simulink model "ADAS_Main"  (R2026a)
settings: Solver=FixedStepDiscrete  StopTime=5
InitFcn:
  | createLidarActorProfiles;
model workspace (MAT data in the model file):
  firstWarning = 1
  originalScenarioChecksum = '71EAF3DF157DF5A35F75811B676F8B0F'
undefined symbols (not defined in the file): driving, matlabshared
libraries: drivingscenarioandsensors x3, lidarlib x1
(part 5 of 6)

== matlab function ADAS_Main/Behavior_Planning/Plan_Feasibility ==
  data: CandV input; CandFeasStatus output; CandCurv input; CandValid input; CandFeasible output; CandViolFlags output; CandPeakAy output; CandKappa output; CandPeakDemand output; CandExceedsEmergency output; CandPeakLatJerk output; CandExceedsLateralJerk output; HardValid output; NormalValid output; ConfigFault output
function [CandFeasStatus, CandFeasible, CandViolFlags, CandPeakAy, CandKappa, ...
          CandPeakDemand, CandExceedsEmergency, CandPeakLatJerk, ...
          CandExceedsLateralJerk, HardValid, NormalValid, ConfigFault] = ...
    Plan_Feasibility(CandV, CandCurv, CandValid) %#codegen
%PLAN_FEASIBILITY  Planning Stage 2 - DYNAMIC FEASIBILITY ONLY.
%
%   Determines whether each of the 35 Stage-1 candidates is dynamically
%   feasible. It performs NO collision checking, NO risk evaluation, NO
%   manoeuvre selection and NO planning decision.
%
%   It reads ONLY the candidate trajectory and configured vehicle/ODD
%   parameters. No TrackState, TrackID, TrackCov, TrackAttributes, Verdict3,
%   RiskValid, M_adm or Bind is available to it - that independence is
%   structural, not conventional, because no such input is wired.
%
%   NOTE ON HORIZONS: every equation below is evaluated per SAMPLE and none
%   requires a time value, so Stage 2 introduces NO horizon grid of its own.
%   It consumes the existing Stage-1 35 x 11 sample structure unchanged.
%
% HARD constraints - these and only these reject a candidate
%   H2   |kappa| <= KAPPA_MAX                      once per candidate
%   H3a  ax      <= A_ACC_MAX                      once per candidate
%   H4'  sqrt(ax^2 + ay^2) <= MU_LO*G              ALL 11 samples
%        with ay = v^2 * kappa      (no division by v anywhere)
%
% NORMAL constraints - DIAGNOSTIC ONLY, never reject
%   N1   |ay| <= A_Y_NORMAL
%   N2   |ax| <= A_BRK_NORMAL       not evaluated while A_BRK_NORMAL is unset
%
% DIAGNOSTIC ONLY - never reject, never alter CandFeasStatus
%   lateral jerk  j_y = 2*v*ax*kappa      (trajectory diagnostic; NO claim of
%                 regulatory equivalence to a half-second moving average)
%   emergency     |ax| >= EmergencyBoundary
%
% H2 and H3a are evaluated once per candidate because kappa and ax are constant
% by construction in Stage 1 (measured: max |kappa(n+1)-kappa(n)| = 0.000e+00).
% The test suite asserts per-sample evaluation is bit-identical, so the
% assumption is monitored rather than trusted.

%% ---- constants, copied VERBATIM from plan_par.m ------------------------
MAXC = 35;
NH   = 11;
G    = 9.80665;
ACC_TABLE = [-8.0 -5.0 -1.0 0.0 2.0];

% Vehicle geometry (B) and the declared turning assumption (E). KAPPA_MAX is
% DERIVED here with the identical expression used in plan_par.m rather than
% written as a decimal literal: a 15-digit literal does not round-trip and
% would differ from plan_par.m by 1 ulp, breaking the single-source discipline.
% Deriving it makes the two bit-identical by construction.
L_WB   = 2.80;                   % B  wheelbase [m]
W_VEH  = 1.80;                   % B  overall body width [m]
FO_VEH = 0.90;                   % B  front overhang [m]
R_WALL_DECLARED = 6.0;           % E  DECLARED RESEARCH-MODEL ASSUMPTION [m]
R_r       = sqrt(R_WALL_DECLARED^2 - (L_WB + FO_VEH)^2) - W_VEH/2;   % F
KAPPA_MAX = 1/R_r;                                                    % F
A_ACC_MAX = 2.0;                 % E  DECLARED RESEARCH-MODEL ASSUMPTION
MU_LO     = 0.50;                % E  DECLARED RESEARCH-MODEL ASSUMPTION

A_Y_NORMAL        = 3.0;         % C  provisional, UN R79 - diagnostic only
A_BRK_NORMAL      = NaN;         %    UNRESOLVED / non-blocking
LateralJerkNormal = 5.0;         % C  provisional, UN R79 - diagnostic only
EmergencyBoundary = 6.0;         % C  UN R13-H - diagnostic only

%% ---- parameter validity: gate on the FLAG, never on the value ----------
% The only permitted read of a parameter that may be unset is the finiteness
% and positivity test that establishes its invalidity. No NaN ever reaches a
% constraint comparison, because every comparison is guarded by its flag.
MU_VALID           = isfinite(MU_LO)             && (MU_LO > 0);
KAPPA_VALID        = isfinite(KAPPA_MAX)         && (KAPPA_MAX > 0);
AACC_VALID         = isfinite(A_ACC_MAX)         && (A_ACC_MAX > 0);
AY_NORMAL_VALID    = isfinite(A_Y_NORMAL)        && (A_Y_NORMAL > 0);
ABRK_NORMAL_VALID  = isfinite(A_BRK_NORMAL)      && (A_BRK_NORMAL > 0);
JERK_NORMAL_VALID  = isfinite(LateralJerkNormal) && (LateralJerkNormal > 0);

HardValid   = MU_VALID && KAPPA_VALID && AACC_VALID;
NormalValid = AY_NORMAL_VALID && ABRK_NORMAL_VALID;
ConfigFault = ~HardValid;        % NORMAL validity never contributes

MU_LIMIT = 0;
if MU_VALID
    MU_LIMIT = MU_LO*G;
end

%% ---- outputs preallocated ---------------------------------------------
CandFeasStatus         = zeros(MAXC,1,'int8');
CandFeasible           = false(MAXC,1);
CandViolFlags          = zeros(MAXC,1,'uint8');
CandPeakAy             = zeros(MAXC,1);
CandKappa              = zeros(MAXC,1);
CandPeakDemand         = zeros(MAXC,1);
CandExceedsEmergency   = false(MAXC,1);
CandPeakLatJerk        = zeros(MAXC,1);
CandExceedsLateralJerk = false(MAXC,1);

for c = 1:MAXC
    if ~CandValid(c)
        % not generated: definitively not executable; all diagnostics zero
        CandFeasStatus(c) = int8(2);
        CandViolFlags(c)  = uint8(1);
        if ~HardValid
            CandViolFlags(c) = bitor(CandViolFlags(c), uint8(64));
        end
        continue
    end

    ia = floor((c-1)/7) + 1;
    ax = ACC_TABLE(ia);
    k  = CandCurv(c,1);
    CandKappa(c) = k;

    peakAy = 0; peakDem = 0; peakJerk = 0;
    h4ok = true; n1ok = true;
    for n = 1:NH
        v  = CandV(c,n);
        kk = CandCurv(c,n);
        ay = v*v*kk;
        if abs(ay) > peakAy, peakAy = abs(ay); end
        dem = sqrt(ax*ax + ay*ay);
        if dem > peakDem, peakDem = dem; end
        jy = 2*v*ax*kk;
        if abs(jy) > peakJerk, peakJerk = abs(jy); end
        if MU_VALID && dem > MU_LIMIT,        h4ok = false; end
        if AY_NORMAL_VALID && abs(ay) > A_Y_NORMAL, n1ok = false; end
    end
    CandPeakAy(c)      = peakAy;
    CandPeakDemand(c)  = peakDem;
    CandPeakLatJerk(c) = peakJerk;

    h2ok = true;
    if KAPPA_VALID && abs(k) > KAPPA_MAX, h2ok = false; end
    h3ok = true;
    if AACC_VALID && ax > A_ACC_MAX, h3ok = false; end
    n2ok = true;
    if ABRK_NORMAL_VALID && abs(ax) > A_BRK_NORMAL, n2ok = false; end

    f = uint8(0);
    if KAPPA_VALID && ~h2ok, f = bitor(f,uint8(2));  end
    if AACC_VALID  && ~h3ok, f = bitor(f,uint8(4));  end
    if MU_VALID    && ~h4ok, f = bitor(f,uint8(8));  end
    if AY_NORMAL_VALID   && ~n1ok, f = bitor(f,uint8(16)); end
    if ABRK_NORMAL_VALID && ~n2ok, f = bitor(f,uint8(32)); end
    if ~HardValid,                 f = bitor(f,uint8(64)); end
    CandViolFlags(c) = f;

    % NORMAL bits 16/32 and the diagnostics below appear NOWHERE in evalFail.
    evalFail = (KAPPA_VALID && ~h2ok) || (AACC_VALID && ~h3ok) || (MU_VALID && ~h4ok);
    if evalFail
        CandFeasStatus(c) = int8(2);
    elseif HardValid
        CandFeasStatus(c) = int8(1);
    else
        CandFeasStatus(c) = int8(0);
    end

    if JERK_NORMAL_VALID && peakJerk > LateralJerkNormal
        CandExceedsLateralJerk(c) = true;
    end
    if abs(ax) >= EmergencyBoundary
        CandExceedsEmergency(c) = true;
    end
end

CandFeasible = (CandFeasStatus == int8(1));
end

== matlab function ADAS_Main/Behavior_Planning/Plan_Envelopes ==
  data: CandX input; CandSpatialStatus output; CandY input; CandCurv input; CandFeasStatus input; TrackState input; TrackAttributes input; TrackStatus input; TrackID input; CandMinSeparation output; CandFirstConflictH output; CandConflictCount output; CandConflictIDs output; CandSpatialFlags output; NumSpatialFeasible output
function [CandSpatialStatus, CandMinSeparation, CandFirstConflictH, ...
          CandConflictCount, CandConflictIDs, CandSpatialFlags, ...
          NumSpatialFeasible] = Plan_Envelopes( ...
          CandX, CandY, CandCurv, CandFeasStatus, ...
          TrackState, TrackAttributes, TrackStatus, TrackID) %#codegen
%PLAN_ENVELOPES  Planning Stage 3 - SPATIAL / ENVELOPE FEASIBILITY ONLY.
%
%   Answers: does each Stage-2 FEASIBLE candidate stay spatially clear of the
%   predicted tracked environment over the approved horizons?
%
%   It is NOT risk scoring, NOT manoeuvre selection, NOT behaviour or intention
%   inference, NOT TTC, and NOT a second fusion stage. It produces per-candidate
%   spatial evidence; Risk and Stage 4 consume it. TrackCov is deliberately NOT
%   an input - uncertainty stays in the Risk Engine.
%
%   STATELESS. No Unit Delay, no Memory, no persistent. Every cycle evaluates
%   all current candidates against the current environment.
%
% PREDICTION (approved): Prediction_Horizons propagates the mean with a constant
%   velocity model, so the predicted mean is exactly p + v*h. Verified against
%   the logged trkPred over 51 frames x 7 horizons at max difference 0.000e+00.
%   TrackPredictions is therefore NOT exposed from Tracking and no new Planning
%   input is required. The test suite asserts this identity permanently.
%
% LIMITATION, recorded deliberately: Stage 3 is SAMPLED spatial feasibility at
%   7 horizons, NOT a continuous collision guarantee. Between consecutive
%   samples 0.5 s elapses, during which a 15 m/s closing speed covers 7.5 m.
%   Swept-volume checking is not implemented. This is not minimised.

%% ---- constants, copied VERBATIM from plan_par.m ------------------------
MAXC = 35; MAXT = 512; MAXREJ = 32; NHS = 7;
HS   = [0.5 1.0 1.5 2.0 3.0 4.0 5.0];
HIDX = [2 3 4 5 7 9 11];

EGO_BOX_XMIN = -1.00; EGO_BOX_XMAX = 3.70;
EGO_BOX_YMIN = -0.90; EGO_BOX_YMAX = 0.90;
PLANNING_EGO_COLLISION_MARGIN = 0.0;
OBJECT_ORIENTATION_SPEED_THRESHOLD = 1.0;
SEP_NOOBJ = 1000.0;

% ego collision box, expressed about the rear-axle reference point
EGO_CX = 0.5*(EGO_BOX_XMIN + EGO_BOX_XMAX);                            % 1.35
EGO_HX = 0.5*(EGO_BOX_XMAX - EGO_BOX_XMIN) + PLANNING_EGO_COLLISION_MARGIN;
EGO_HY = 0.5*(EGO_BOX_YMAX - EGO_BOX_YMIN) + PLANNING_EGO_COLLISION_MARGIN;

%% ---- outputs preallocated ---------------------------------------------
CandSpatialStatus  = zeros(MAXC,1,'int8');
CandMinSeparation  = SEP_NOOBJ*ones(MAXC,NHS);
CandFirstConflictH = zeros(MAXC,1,'uint8');
CandConflictCount  = zeros(MAXC,1,'uint16');
CandConflictIDs    = zeros(MAXC,MAXREJ,'uint32');
CandSpatialFlags   = zeros(MAXC,1,'uint8');
NumSpatialFeasible = uint16(0);

seen = false(MAXT,1);

for c = 1:MAXC
    % Stage-2 rejection is ABSORBING: a candidate the vehicle cannot execute
    % can never become feasible through good clearance.
    if CandFeasStatus(c) ~= int8(1)
        CandSpatialStatus(c) = int8(2);
        CandSpatialFlags(c)  = uint8(1);
        continue
    end

    for t = 1:MAXT, seen(t) = false; end
    nConf = uint16(0); overflow = false;
    anyOverlap = false; anyUnknown = false;
    firstH = uint8(0);
    fUnusable = false; fDims = false; fCoast = false;

    for hi = 1:NHS
        n = HIDX(hi);
        h = HS(hi);
        kap = CandCurv(c,n);
        cx  = CandX(c,n);
        cy  = CandY(c,n);
        % ego heading on the constant-curvature arc: kap*x = sin(psi),
        % 1 - kap*y = cos(psi). Exact, and atan2(0,1) = 0 when kap = 0.
        psi = atan2(kap*cx, 1 - kap*cy);
        cp  = cos(psi); sp = sin(psi);
        eEx = cp; eEy = sp;                 % ego longitudinal axis
        fEx = -sp; fEy = cp;                % ego lateral axis
        ecx = cx + EGO_CX*cp;               % ego box centre
        ecy = cy + EGO_CX*sp;

        minsep = SEP_NOOBJ;
        for t = 1:MAXT
            if TrackStatus(t) == 0
                continue                     % FREE slot: not an object
            end
            if TrackAttributes(t,1) ~= 1
                anyUnknown = true; fUnusable = true; continue
            end
            Lo = TrackAttributes(t,2);
            Wo = TrackAttributes(t,3);
            if ~isfinite(Lo) || ~isfinite(Wo) || Lo <= 0 || Wo <= 0
                anyUnknown = true; fDims = true; continue
            end
            px = TrackState(t,1); py = TrackState(t,2);
            vx = TrackState(t,3); vy = TrackState(t,4);
            if ~isfinite(px) || ~isfinite(py) || ~isfinite(vx) || ~isfinite(vy)
                anyUnknown = true; continue
            end
            ocx = px + vx*h;                 % approved prediction: p + v*h
            ocy = py + vy*h;
            if ~isfinite(ocx) || ~isfinite(ocy)
                anyUnknown = true; continue
            end
            if TrackStatus(t) == 3
                fCoast = true;
            end

            sv = sqrt(vx*vx + vy*vy);
            if sv > OBJECT_ORIENTATION_SPEED_THRESHOLD
                oEx = vx/sv; oEy = vy/sv;    % oriented along velocity
            else
                oEx = 1.0;  oEy = 0.0;       % axis-aligned fallback
            end
            oFx = -oEy; oFy = oEx;
            ohx = 0.5*Lo; ohy = 0.5*Wo;

            dx = ocx - ecx; dy = ocy - ecy;

            % separating-axis test over the 4 box axes
            sep = -realmax;
            for ax = 1:4
                if ax == 1
                    axx = eEx; axy = eEy;
                elseif ax == 2
                    axx = fEx; axy = fEy;
                elseif ax == 3
                    axx = oEx; axy = oEy;
                else
                    axx = oFx; axy = oFy;
                end
                rE = abs(EGO_HX*(axx*eEx + axy*eEy)) + abs(EGO_HY*(axx*fEx + axy*fEy));
                rO = abs(ohx *(axx*oEx + axy*oEy)) + abs(ohy *(axx*oFx + axy*oFy));
                d  = abs(dx*axx + dy*axy);
                g  = d - (rE + rO);
                if g > sep, sep = g; end
            end

            if sep < minsep, minsep = sep; end

            if sep <= 0
                anyOverlap = true;
                if firstH == uint8(0), firstH = uint8(hi); end
                if ~seen(t)
                    seen(t) = true;
                    nConf = nConf + uint16(1);
                    if nConf <= uint16(MAXREJ)
                        CandConflictIDs(c,double(nConf)) = TrackID(t);
                    else
                        overflow = true;
                    end
                end
            end
        end
        CandMinSeparation(c,hi) = minsep;
    end

    CandConflictCount(c)  = nConf;           % ALL conflicts, never truncated
    CandFirstConflictH(c) = firstH;

    f = uint8(0);
    if anyOverlap, f = bitor(f,uint8(2));  end
    if fUnusable,  f = bitor(f,uint8(4));  end
    if fDims,      f = bitor(f,uint8(8));  end
    if fCoast,     f = bitor(f,uint8(16)); end
    if overflow,   f = bitor(f,uint8(32)); end
    CandSpatialFlags(c) = f;

    % A definite overlap is certifiable even when unknowns are present, so
    % INFEASIBLE takes precedence over UNKNOWN. Uncertainty is never converted
    % into safety: an unusable track leaves the candidate UNKNOWN, not FEASIBLE.
    if anyOverlap
        CandSpatialStatus(c) = int8(2);
    elseif anyUnknown
        CandSpatialStatus(c) = int8(0);
    else
        CandSpatialStatus(c) = int8(1);
        NumSpatialFeasible = NumSpatialFeasible + uint16(1);
    end
end
end

== matlab function ADAS_Main/Behavior_Planning/Plan_Evaluate ==
  data: CandY input; CandAdmissible output; CandV input; CandFeasStatus input; CandSpatialStatus input; CandMinSeparation input; EgoKinematics input; CandWorstClearance output; CandLateralOffset output; CandSpeedDelta output; CandRejectReason output
function [CandAdmissible, CandWorstClearance, CandLateralOffset, ...
          CandSpeedDelta, CandRejectReason] = Plan_Evaluate( ...
          CandY, CandV, CandFeasStatus, CandSpatialStatus, ...
          CandMinSeparation, EgoKinematics) %#codegen
%PLAN_EVALUATE  Planning Stage 4a - per-candidate comparative metrics.
%
%   Computes the quantities the lexicographic selector needs. It performs NO
%   selection, NO ranking, NO risk evaluation, NO TTC, NO intention inference
%   and NO behaviour classification.
%
%   STATELESS. No Unit Delay, no Memory, no persistent.
%
%   HARD GATE, and the only one:
%       admissible(c) = (CandFeasStatus(c) == 1) AND (CandSpatialStatus(c) == 1)
%   A candidate must pass BOTH Stage 2 and Stage 3 to be selectable. Note that
%   NumFeasible (Stage-2 count) is NOT the number of selectable candidates.
%
%   ICE and Risk are deliberately absent from this block. They are indexed by
%   sector x horizon, not by candidate, and are never reinterpreted as
%   candidate scores.

MAXC = 35; NHS = 7;

CandAdmissible     = false(MAXC,1);
CandWorstClearance = zeros(MAXC,1);
CandLateralOffset  = zeros(MAXC,1);
CandSpeedDelta     = zeros(MAXC,1);
CandRejectReason   = zeros(MAXC,1,'uint8');

v0 = EgoKinematics(1);
if ~isfinite(v0), v0 = 0; end
if v0 < 0, v0 = 0; end

for c = 1:MAXC
    % terminal-sample metrics are defined for every candidate, admissible or not
    CandLateralOffset(c) = CandY(c,11);
    CandSpeedDelta(c)    = abs(CandV(c,11) - v0);

    wc = CandMinSeparation(c,1);
    for h = 2:NHS
        if CandMinSeparation(c,h) < wc, wc = CandMinSeparation(c,h); end
    end
    CandWorstClearance(c) = wc;

    adm = (CandFeasStatus(c) == int8(1)) && (CandSpatialStatus(c) == int8(1));
    CandAdmissible(c) = adm;

    % rejection reason, retained for ALL 35 candidates and never truncated.
    % 'not selected' (8) is applied later by Plan_Select; here an admissible
    % candidate carries 0 until selection resolves it.
    if CandFeasStatus(c) ~= int8(1)
        CandRejectReason(c) = uint8(1);          % Stage-2 rejection
    elseif CandSpatialStatus(c) == int8(2)
        CandRejectReason(c) = uint8(2);          % Stage-3 overlap
    elseif CandSpatialStatus(c) == int8(0)
        CandRejectReason(c) = uint8(4);          % Stage-3 unknown
    else
        CandRejectReason(c) = uint8(0);
    end
end
end

== matlab function ADAS_Main/Behavior_Planning/Plan_Select ==
  data: CandAdmissible input; TrajX output; CandWorstClearance input; CandLateralOffset input; CandSpeedDelta input; CandRejectReason input; CandX input; CandY input; CandV input; CandCurv input; CandFeasStatus input; CandSpatialStatus input; TrackStatus input; ConfigFault input; RiskValid input; TrajY output; TrajV output; TrajCurv output; TrajValid output; ManoeuvreLabel output; FallbackActive output; NumFeasible output; NumClear output; NumTracksEvaluated output; RejectIDs output; PlanStale output; NoFeasibleReason output; RejectOverflow output; SelectedCandidate output; CandRejectReasonOut output
function [TrajX, TrajY, TrajV, TrajCurv, TrajValid, ManoeuvreLabel, ...
          FallbackActive, NumFeasible, NumClear, NumTracksEvaluated, ...
          RejectIDs, PlanStale, NoFeasibleReason, RejectOverflow, ...
          SelectedCandidate, CandRejectReasonOut] = Plan_Select( ...
          CandAdmissible, CandWorstClearance, CandLateralOffset, ...
          CandSpeedDelta, CandRejectReason, ...
          CandX, CandY, CandV, CandCurv, ...
          CandFeasStatus, CandSpatialStatus, TrackStatus, ...
          ConfigFault, RiskValid) %#codegen
%PLAN_SELECT  Planning Stage 4b - lexicographic selection and public outputs.
%
%   STATELESS. No Unit Delay, no Memory, no persistent, no previous-selection
%   state. Every cycle selects from the CURRENT admissible set only, so an
%   ongoing manoeuvre has no privileged status: if the candidate selected last
%   cycle is no longer admissible it simply is not in the set. There is no
%   overtaking mode, no abort mode, no "obstacle handled" state, and no
%   primary-object priority.
%
% HARD GATE - the only selection path
%   admissible(c) = (CandFeasStatus(c)==1) AND (CandSpatialStatus(c)==1)
%   INVARIANT: TrajValid == true  =>  both hold for the selected candidate.
%
% LEXICOGRAPHIC ORDER with tolerance bands (no weighted sum, no score)
%   KEY 1  CandWorstClearance  larger preferred   band BAND_CLEAR = 0.05 m
%   KEY 2  |CandLateralOffset| smaller preferred  band BAND_LAT   = 0.50 m
%   KEY 3  CandSpeedDelta      smaller preferred  band BAND_SPD   = 2.50 m/s
%   TIE    lowest candidate index
%   CandProgress is NOT a ranking key: forward distance may never buy down
%   clearance.
%
% ZERO-FEASIBLE STATE
%   FallbackActive = true means "Planning has no admissible trajectory and is
%   NOT commanding one". It does NOT mean emergency braking is commanded. No
%   fallback manoeuvre exists in the current candidate library and none is
%   fabricated here.

MAXC = 35; NH = 11; MAXREJ = 32; MAXT = 512;

% tolerance bands, copied VERBATIM from plan_par.m
BAND_CLEAR = 0.05;
BAND_LAT   = 0.50;
BAND_SPD   = 2.50;

TrajX  = zeros(NH,1); TrajY = zeros(NH,1);
TrajV  = zeros(NH,1); TrajCurv = zeros(NH,1);
TrajValid          = false;
ManoeuvreLabel     = uint8(0);
FallbackActive     = false;
NumFeasible        = uint16(0);
NumClear           = uint16(0);
NumTracksEvaluated = uint16(0);
RejectIDs          = zeros(MAXREJ,1,'uint32');
PlanStale          = false;
NoFeasibleReason   = uint8(0);
RejectOverflow     = false;
SelectedCandidate  = uint8(0);
CandRejectReasonOut = CandRejectReason;

%% ---- counts ------------------------------------------------------------
nS2 = uint16(0); nS3 = uint16(0);
for c = 1:MAXC
    if CandFeasStatus(c) == int8(1),    nS2 = nS2 + uint16(1); end
    if CandSpatialStatus(c) == int8(1), nS3 = nS3 + uint16(1); end
end
NumFeasible = nS2;      % Stage-2 count. NOT the number of selectable candidates.
NumClear    = nS3;      % Stage-3 count.
nT = uint16(0);
for t = 1:MAXT
    if TrackStatus(t) ~= 0, nT = nT + uint16(1); end
end
NumTracksEvaluated = nT;

%% ---- PlanStale: input usability only, NOT "nothing is feasible" -------
% AdmVacuous is deliberately excluded: it is an ICE scene state, not a
% statement that a Planning input is unusable.
PlanStale = ConfigFault || ~RiskValid;

%% ---- KEY 1: worst-case clearance, larger preferred ---------------------
nAdm = 0; best1 = 0;
for c = 1:MAXC
    if CandAdmissible(c)
        if nAdm == 0 || CandWorstClearance(c) > best1, best1 = CandWorstClearance(c); end
        nAdm = nAdm + 1;
    end
end

if nAdm == 0
    FallbackActive = true;
    TrajValid      = false;          % never true without an admissible candidate
    ManoeuvreLabel = uint8(0);
    if PlanStale
        NoFeasibleReason = uint8(8);                 % upstream invalid
    elseif nS2 == uint16(0)
        NoFeasibleReason = uint8(1);                 % all rejected at Stage 2
    elseif nS2 == uint16(MAXC)
        NoFeasibleReason = uint8(2);                 % all rejected at Stage 3
    else
        NoFeasibleReason = uint8(4);                 % mixed
    end
else
    keep1 = false(MAXC,1);
    for c = 1:MAXC
        if CandAdmissible(c) && CandWorstClearance(c) >= best1 - BAND_CLEAR
            keep1(c) = true;
        end
    end

    % KEY 2: |lateral offset|, smaller preferred
    best2 = 0; first = true;
    for c = 1:MAXC
        if keep1(c)
            a = abs(CandLateralOffset(c));
            if first || a < best2, best2 = a; first = false; end
        end
    end
    keep2 = false(MAXC,1);
    for c = 1:MAXC
        if keep1(c) && abs(CandLateralOffset(c)) <= best2 + BAND_LAT
            keep2(c) = true;
        end
    end

    % KEY 3: terminal-speed disturbance, smaller preferred
    best3 = 0; first = true;
    for c = 1:MAXC
        if keep2(c)
            if first || CandSpeedDelta(c) < best3, best3 = CandSpeedDelta(c); first = false; end
        end
    end
    keep3 = false(MAXC,1);
    for c = 1:MAXC
        if keep2(c) && CandSpeedDelta(c) <= best3 + BAND_SPD
            keep3(c) = true;
        end
    end

    % TIE: lowest candidate index
    sel = 0;
    for c = 1:MAXC
        if keep3(c), sel = c; break; end
    end

    SelectedCandidate = uint8(sel);
    ManoeuvreLabel    = uint8(sel);          % the candidate index IS the label
    TrajValid         = true;
    FallbackActive    = false;
    for n = 1:NH
        TrajX(n)    = CandX(sel,n);
        TrajY(n)    = CandY(sel,n);
        TrajV(n)    = CandV(sel,n);
        TrajCurv(n) = CandCurv(sel,n);
    end
    CandRejectReasonOut(sel) = uint8(0);
end

%% ---- rejection bookkeeping --------------------------------------------
% every non-selected candidate carries a reason; admissible-but-not-selected
% is reason 8. Nothing is silently discarded.
for c = 1:MAXC
    if uint8(c) ~= SelectedCandidate && CandRejectReasonOut(c) == uint8(0)
        CandRejectReasonOut(c) = uint8(8);
    end
end
nRej = 0;
for c = 1:MAXC
    if CandRejectReasonOut(c) ~= uint8(0)
        nRej = nRej + 1;
        if nRej <= MAXREJ
            RejectIDs(nRej) = uint32(c);     % ascending, deterministic
        else
            RejectOverflow = true;
        end
    end
end
end

== matlab function ADAS_Main/Behavior_Planning/Plan_Continuity ==
  data: CandAdmissible input; TrajX output; CandWorstClearance input; CandX input; CandY input; CandV input; CandCurv input; Challenger input; CandRejectReason input; NumFeasible_in input; NumClear_in input; NumTracksEvaluated_in input; PlanStale_in input; PrevSelected_in input uint8 size=1; SelectionAge_in input uint16 size=1; TrajY output; TrajV output; TrajCurv output; TrajValid output; ManoeuvreLabel output; FallbackActive output; NumFeasible output; NumClear output; NumTracksEvaluated output; RejectIDs output; PlanStale output; PrevSelected_out output; SelectionAge_out output; ContinuityHeld output; SwitchReason output
function [TrajX, TrajY, TrajV, TrajCurv, TrajValid, ManoeuvreLabel, ...
          FallbackActive, NumFeasible, NumClear, NumTracksEvaluated, ...
          RejectIDs, PlanStale, ...
          PrevSelected_out, SelectionAge_out, ContinuityHeld, SwitchReason] = ...
    Plan_Continuity( ...
          CandAdmissible, CandWorstClearance, CandX, CandY, CandV, CandCurv, ...
          Challenger, CandRejectReason, NumFeasible_in, NumClear_in, ...
          NumTracksEvaluated_in, PlanStale_in, PrevSelected_in, SelectionAge_in) %#codegen
%PLAN_CONTINUITY  Planning Stage 5 - temporal continuity / hysteresis.
%
%   Prefers the previously selected candidate while it REMAINS ADMISSIBLE and
%   the current challenger is not materially better. It performs no evaluation,
%   no ranking, no risk assessment and no object reasoning.
%
%   SCENARIO INDEPENDENT BY CONSTRUCTION. Its entire input set is an
%   admissibility mask, one scalar metric per candidate, the challenger index
%   and its own previous index. It cannot see actor IDs, actor counts, object
%   classes, coordinates, road geometry, timing or ego speed, so it cannot
%   contain scenario-specific logic. There is no overtaking mode, no abort
%   mode, no object priority and no "obstacle handled" state.
%
% SAFETY PRIORITY, absolute
%   HARD SAFETY FEASIBILITY  >  TEMPORAL CONTINUITY  >  SOFT PREFERENCE
%   The previous candidate is re-gated against the CURRENT admissibility mask
%   every cycle. Continuity can only ever choose among candidates that are
%   admissible NOW, so it can never make an inadmissible candidate selectable.
%
% NO minimum hold time. NO N-cycle persistence. NO switching penalty or score.
% NO hidden delay. A materially safer challenger replaces the previous
% candidate on the SAME cycle, and an inadmissible previous candidate is
% abandoned on the SAME cycle.

MAXC = 35; NH = 11; MAXREJ = 32;
SWITCH_MARGIN = 0.05;            % copied VERBATIM from plan_par.m

TrajX = zeros(NH,1); TrajY = zeros(NH,1);
TrajV = zeros(NH,1); TrajCurv = zeros(NH,1);
TrajValid          = false;
ManoeuvreLabel     = uint8(0);
FallbackActive     = false;
NumFeasible        = NumFeasible_in;
NumClear           = NumClear_in;
NumTracksEvaluated = NumTracksEvaluated_in;
RejectIDs          = zeros(MAXREJ,1,'uint32');
PlanStale          = PlanStale_in;
ContinuityHeld     = false;
SwitchReason       = uint8(0);
SelectionAge_out   = uint16(0);

%% ---- previous selection, re-gated against the CURRENT mask -------------
prev = PrevSelected_in;
if PlanStale_in
    prev = uint8(0);                 % never rest continuity on unusable input
    SwitchReason = uint8(8);
end
prevOK = false;
if prev ~= uint8(0) && prev <= uint8(MAXC)
    if CandAdmissible(double(prev))
        prevOK = true;               % admissible THIS cycle, not last cycle
    end
end

%% ---- continuity decision -----------------------------------------------
% SWITCH_MARGIN = 0 disables hysteresis entirely, so Stage 5 reproduces
% Stage-4 output bit-identically. The guard is required because Stage 4's
% winner is the LEXICOGRAPHIC winner, which may carry lower clearance than an
% admissible previous candidate; a clearance-only test at margin 0 would still
% retain the previous one and would not reproduce Stage 4.
sel = Challenger;
if (SWITCH_MARGIN > 0) && prevOK
    takeChallenger = false;
    if Challenger ~= uint8(0)
        if CandWorstClearance(double(Challenger)) > ...
           CandWorstClearance(double(prev)) + SWITCH_MARGIN
            takeChallenger = true;   % materially better
        end
    end
    if takeChallenger
        sel = Challenger;
        SwitchReason = uint8(2);
    else
        sel = prev;                  % retained; it passed the gate this cycle
        ContinuityHeld = true;
    end
else
    if SwitchReason == uint8(0)
        if prev == uint8(0)
            SwitchReason = uint8(4); % no previous selection
        elseif ~prevOK
            SwitchReason = uint8(1); % previous no longer admissible
        else
            SwitchReason = uint8(2); % challenger taken (hysteresis disabled)
        end
    end
end

%% ---- emit ---------------------------------------------------------------
rr = CandRejectReason;
if sel ~= uint8(0)
    % defensive: emit ONLY a candidate that passes the current hard gate
    if ~CandAdmissible(double(sel))
        sel = uint8(0);
    end
end

if sel == uint8(0)
    TrajValid        = false;
    FallbackActive   = true;
    ManoeuvreLabel   = uint8(0);
    PrevSelected_out = uint8(0);
    SelectionAge_out = uint16(0);
    for c = 1:MAXC
        if rr(c) == uint8(0), rr(c) = uint8(8); end
    end
else
    TrajValid      = true;
    FallbackActive = false;
    ManoeuvreLabel = sel;
    for n = 1:NH
        TrajX(n)    = CandX(double(sel),n);
        TrajY(n)    = CandY(double(sel),n);
        TrajV(n)    = CandV(double(sel),n);
        TrajCurv(n) = CandCurv(double(sel),n);
    end
    PrevSelected_out = sel;
    if sel == PrevSelected_in && ~PlanStale_in
        SelectionAge_out = SelectionAge_in + uint16(1);
    else
        SelectionAge_out = uint16(1);
    end
    % reject bookkeeping follows the ACTUAL selection, not Stage-4's proposal
    if Challenger ~= uint8(0) && Challenger ~= sel
        rr(double(Challenger)) = uint8(8);
    end
    rr(double(sel)) = uint8(0);
end

nRej = 0;
for c = 1:MAXC
    if rr(c) ~= uint8(0)
        nRej = nRej + 1;
        if nRej <= MAXREJ
            RejectIDs(nRej) = uint32(c);
        end
    end
end
end

== matlab function ADAS_Main/Radar_Perception/Radar_Feature_Extraction/Extract_Radar_Features ==
  data: u input; RadarFeatures output
function RadarFeatures = fcn(u)

N = 50;

RadarFeatures = zeros(N,8);

for i = 1:N
    RadarFeatures(i,1) = double(i <= u.NumDetections);
    RadarFeatures(i,2:7) = double(u.Detections(i).Measurement);
    RadarFeatures(i,8) = double(u.Detections(i).ObjectAttributes.SNR);
end

== matlab function ADAS_Main/Behavior_Controller/Ctrl_Lateral ==
  data: TrajCurv input; SteerCmd output; TrajValid input; EgoKinematics input; CmdValid output; CtrlCurvatureRef output; CtrlState output
function [SteerCmd, CmdValid, CtrlCurvatureRef, CtrlState] = ...
    Ctrl_Lateral(TrajCurv, TrajValid, EgoKinematics) %#codegen
%CTRL_LATERAL  Controller Stage C1 - LATERAL FEEDFORWARD ONLY.
%
%   Converts the curvature of the Planning-selected trajectory into a
%   front-road-wheel-equivalent steering command. It does NOTHING else.
%
% NOT IMPLEMENTED IN C1, BY AUTHORIZATION
%   no longitudinal control, no feedback of any kind (k_y, k_psi, k_v,
%   Stanley, Pure Pursuit, LQR, MPC), no steering-rate limit, no actuator
%   model, no braking or fallback policy, no PlanStale handling, no vehicle
%   dynamics. There is NO state: no persistent, no Unit Delay, no Memory.
%   The block is a pure function of its inputs.
%
% SCENARIO INDEPENDENT BY CONSTRUCTION
%   The entire input set is one curvature array, one boolean, and two ego
%   self-kinematic scalars. The block never receives actor IDs, track IDs,
%   object classes, actor counts, coordinates, road or intersection geometry,
%   lane boundaries or scenario timing, so it cannot contain scenario-specific
%   logic. EgoKinematics is accepted to honour the approved C1 interface and
%   is DELIBERATELY NOT READ - see EGO SPEED below.
%
% EGO SPEED
%   The feedforward law depends on curvature and wheelbase ONLY. Speed does
%   not appear in the kinematic bicycle steering relation. EgoKinematics is
%   therefore left unread, which makes independence from the 15 m/s fixture
%   speed STRUCTURAL rather than a property that has to be tested for.
%
% THE LAW
%   TrajValid == true                        TrajValid == false
%     kappa = TrajCurv(1)                      SteerCmd         = 0
%     d     = atan(L_WB*kappa)                 CmdValid         = false
%     SteerCmd = sat(d, +/-DELTA_MAX)          CtrlCurvatureRef = 0
%     CmdValid = true                          CtrlState        = NO_TRAJECTORY
%     CtrlCurvatureRef = kappa                 (NO trajectory element is read)
%     CtrlState = TRACKING
%
% WHY TrajCurv(1)
%   Sample 1 is at arc length s = 0, i.e. AT THE EGO'S OWN POSITION (Stage 1
%   generates the arc from the origin). atan(L*kappa(0)) is therefore the
%   correct instantaneous kinematic feedforward REGARDLESS of whether the
%   curvature profile is constant further along the horizon. The law needs no
%   constancy fallback. Constancy is proved offline over the public
%   Plan_TrajCurv signal instead of being asserted at runtime, because a
%   runtime non-constancy report would need a fifth output and that would
%   exceed the authorized C1 interface.
%
% THE ZERO SENTINEL
%   When TrajValid is false, Planning emits TrajX/Y/V/Curv = zeros(11,1) as a
%   SENTINEL. Those zeros are NOT a straight-path command and NOT a zero-speed
%   command. TrajCurv is read strictly inside the TrajValid branch, so a
%   sentinel - or a NaN/Inf - can never reach an output.
%
% DERIVED INVARIANT (why no NaN guard exists on the valid branch)
%   TrajValid == true implies the candidate passed Stage-2 H2,
%   |kappa| <= KAPPA_MAX. A NaN or Inf curvature fails that comparison and is
%   rejected upstream, so TrajCurv(1) is finite whenever TrajValid is true.
%   No defensive NaN branch is added here: inventing one would mean inventing
%   an emission policy for a state that cannot occur.
%
% SATURATION
%   |kappa| <= KAPPA_MAX is already guaranteed by H2 for any valid trajectory,
%   so the clamp is STRUCTURALLY UNREACHABLE in integration. It is implemented
%   and tested synthetically as a defensive bound, not as an active limiter.

%% ---- parameters ---------------------------------------------------------
% VERBATIM copy of plan_par.m, audited field-by-field by ctrl_c1_tests.m.
% This is the project's established discipline (see the plan_par.m header):
% a Simulink MATLAB Function block requires compile-time constants, so
% Plan_Feasibility.m carries the same verbatim copy and the same audit.
% NOTHING here is a new parameter and NOTHING here is a measured real-vehicle
% value. Planning parameters are NOT modified by C1.
%
%   L_WB, W_VEH, FO_VEH   B  scenario actor self-geometry
%   R_WALL_DECLARED       E  DECLARED RESEARCH-MODEL ASSUMPTION
%   R_r, KAPPA_MAX        F  derived
%   DELTA_MAX             F  derived - the ONLY quantity C1 adds
%
% KAPPA_MAX is DERIVED with the identical expression used in plan_par.m and
% Plan_Feasibility.m rather than written as a decimal literal: a 15-digit
% literal does not round-trip and would differ by 1 ulp, breaking the
% single-source discipline. Deriving it makes all three bit-identical by
% construction, and DELTA_MAX inherits that property.
L_WB   = 2.80;                   % B  wheelbase [m]
W_VEH  = 1.80;                   % B  overall body width [m]
FO_VEH = 0.90;                   % B  front overhang [m]
R_WALL_DECLARED = 6.0;           % E  DECLARED RESEARCH-MODEL ASSUMPTION [m]
R_r       = sqrt(R_WALL_DECLARED^2 - (L_WB + FO_VEH)^2) - W_VEH/2;   % F
KAPPA_MAX = 1/R_r;                                                    % F

% DELTA_MAX is the kinematic-bicycle-equivalent front road wheel angle at the
% declared minimum wall-to-wall turning radius. It is NOT a steering rack
% mechanical limit, NOT a measured value and NOT a manufacturer figure; those
% are different quantities that merely coincide in a kinematic model.
DELTA_MAX = atan(KAPPA_MAX*L_WB);                                     % F [rad]

% CtrlState codes. C1 emits only TRACKING and NO_TRAJECTORY; IDLE and
% STALE_INPUTS are reserved by the approved interface and never emitted here.
ST_NO_TRAJECTORY = uint8(2);
ST_TRACKING      = uint8(1);

%% ---- default emission: the safe, trajectory-free state ------------------
SteerCmd         = 0;
CmdValid         = false;
CtrlCurvatureRef = 0;
CtrlState        = ST_NO_TRAJECTORY;

%% ---- the gate. TrajCurv is read ONLY inside it --------------------------
if TrajValid
    kappa = TrajCurv(1);

    d = atan(L_WB*kappa);
    if d > DELTA_MAX
        d = DELTA_MAX;
    elseif d < -DELTA_MAX
        d = -DELTA_MAX;
    end

    SteerCmd         = d;
    CmdValid         = true;
    CtrlCurvatureRef = kappa;
    CtrlState        = ST_TRACKING;
end

% EgoKinematics is accepted to honour the approved 3-input C1 interface and is
% intentionally never read, anywhere above. That is deliberate: it makes the
% law's independence from ego speed - and therefore from the fixture's
% constant 15 m/s - a STRUCTURAL property rather than a tested one.
end

== matlab function ADAS_Main/Behavior_Controller/Ctrl_Longitudinal ==
  data: TrajV input; AccelCmd output; TrajValid input; EgoKinematics input; CmdValid output; CtrlState output
function [AccelCmd, CmdValid, CtrlState] = ...
    Ctrl_Longitudinal(TrajV, TrajValid, EgoKinematics) %#codegen
%CTRL_LONGITUDINAL  Controller Stage C2 - LONGITUDINAL FEEDFORWARD ONLY.
%
%   Recovers the planned longitudinal acceleration from the trajectory speed
%   profile and emits it as an acceleration demand. It does NOTHING else.
%
% NOT IMPLEMENTED IN C2, BY AUTHORIZATION
%   no feedback of any kind (no P, no PI, no speed error), no rate or jerk
%   limit, no actuator/throttle/brake mapping, no vehicle dynamics, no
%   fallback braking policy, no PlanStale handling, no loop closure.
%   There is NO state: no persistent, no Unit Delay, no Memory, no previous
%   command, no hold timer. The block is a pure function of its inputs.
%
% EGO SPEED IS NOT FEEDBACK
%   EgoKinematics is accepted for interface consistency with C1 and is
%   DELIBERATELY NOT READ. C2 is feedforward only: the command is a property
%   of the planned trajectory alone. Acceleration is likewise NEVER inferred
%   from EgoKinematics. Leaving it unread makes independence from ego speed -
%   and therefore from the fixture's constant 15 m/s - STRUCTURAL.
%
% THE LAW
%   TrajValid == false -> AccelCmd = 0, CmdValid = false, CtrlState = 2,
%                         and TrajV is NEVER indexed.
%   TrajValid == true  -> see SLOPE SELECTION below.
%
% SLOPE SELECTION, and why the naive first interval is not enough
%   Stage 1 builds the speed profile as v = v0 + a*t, FROZEN AT ZERO once
%   t >= v0/|a|. The samples are 0.5 s apart, so a braking candidate that
%   stops inside the first interval leaves TrajV = [v0 0 0 ...] and the naive
%   slope (TrajV(2)-TrajV(1))/0.5 = -2*v0 UNDERSTATES the deceleration. A
%   naive "last interval" rule is worse still: the repeated-zero tail has
%   slope 0, which would report NO braking at all for a full stop.
%
%   Rule 1  first interval positive THROUGHOUT   -> use its slope
%   Rule 2  otherwise, the LAST interval whose BOTH endpoints are > 0
%   Rule 3  otherwise, if TrajV(1) > 0 the stop occurs inside interval 1
%           -> use interval 1's slope, which is a LOWER BOUND on |a|
%   Rule 4  otherwise the vehicle is already at rest -> 0
%
%   Requiring BOTH endpoints > 0 is what keeps the zero tail from ever being
%   selected, so a full-stop trajectory can never be reported as zero or
%   positive acceleration.
%
% [LIMITATION] Rule 3 cannot recover the true deceleration
%   When the stop falls strictly inside the first 0.5 s interval, the true
%   value of a is NOT RECOVERABLE from TrajV: the data only establishes
%   |a| >= v0/0.5. Rule 3 returns that bound, which UNDER-brakes relative to
%   the planned value. This is an information limit of the 0.5 s horizon
%   sampling, not an implementation choice, and it is reported rather than
%   patched: fixing it would need a new Planning output, which is out of
%   C2 scope.
%
% NUMERICAL GUARD
%   A non-finite TrajV on the valid path is refused, not sanitised into a
%   valid command: AccelCmd = 0 with CmdValid = false. The state is
%   UNREACHABLE - Stage-2 H4' evaluates sqrt(ax^2+ay^2) <= MU_LO*G with
%   ay = v^2*kappa over all 11 samples, and a NaN or Inf speed fails that
%   comparison, so the candidate is rejected and TrajValid is false. The
%   guard is therefore defensive only.

%% ---- parameters ---------------------------------------------------------
% VERBATIM copy of the approved single sources, audited field-by-field by
% ctrl_c2_tests.m - the project's established discipline for compile-time
% constants in a MATLAB Function block, identical to Plan_Feasibility.m and
% Ctrl_Lateral.m. NOTHING here is a new parameter. plan_par.m is NOT modified.
%
%   TH_DT      Tier-1 algorithm constant. TH(2)-TH(1) of the Stage-1 horizon
%              grid TH = [0 0.5 1.0 ... 5.0]. NOT a control period: the model
%              cycle is 0.1 s and is deliberately not used here.
%   A_ACC_MAX  plan_par.m PAR.A_ACC_MAX, class E DECLARED RESEARCH-MODEL
%              ASSUMPTION. Applied as an UPPER bound only.
%
% NO BRAKING LIMIT IS APPLIED. A_BRK_NORMAL remains UNRESOLVED and is NOT
% invented here; there is no lower clamp of any kind, and no V_STOP.
NH        = 11;
TH_DT     = 0.5;                 % [s]      Stage-1 horizon sample spacing
A_ACC_MAX = 2.0;                 % [m/s^2]  E  DECLARED RESEARCH-MODEL ASSUMPTION

ST_NO_TRAJECTORY = uint8(2);
ST_TRACKING      = uint8(1);

%% ---- default emission: the safe, trajectory-free state ------------------
AccelCmd  = 0;
CmdValid  = false;
CtrlState = ST_NO_TRAJECTORY;

%% ---- the gate. TrajV is read ONLY inside it -----------------------------
if TrajValid
    % numerical guard, evaluated before any arithmetic uses the data
    allFinite = true;
    for n = 1:NH
        if ~isfinite(TrajV(n))
            allFinite = false;
        end
    end

    if allFinite
        a = 0;
        if TrajV(1) > 0 && TrajV(2) > 0
            a = (TrajV(2) - TrajV(1))/TH_DT;              % Rule 1
        else
            nSel = 0;
            for n = 1:(NH-1)
                if TrajV(n) > 0 && TrajV(n+1) > 0
                    nSel = n;                             % keep the LAST one
                end
            end
            if nSel > 0
                a = (TrajV(nSel+1) - TrajV(nSel))/TH_DT;  % Rule 2
            elseif TrajV(1) > 0
                a = (TrajV(2) - TrajV(1))/TH_DT;          % Rule 3, lower bound
            else
                a = 0;                                    % Rule 4, at rest
            end
        end

        % Approved acceleration envelope, UPPER bound only. Stage-2 H3a
        % already guarantees ax <= A_ACC_MAX for any admissible candidate, so
        % this clamp is structurally unreachable in integration and exists as
        % a defensive bound, exactly as DELTA_MAX does in C1.
        if a > A_ACC_MAX
            a = A_ACC_MAX;
        end

        AccelCmd  = a;
        CmdValid  = true;
        CtrlState = ST_TRACKING;
    end
end

% EgoKinematics is accepted to honour the approved 3-input C2 interface and is
% intentionally never read, anywhere above.
end

== matlab function ADAS_Main/LiDAR_Perception/LiDAR_Ground_Segmentation/Ground_Segmentation ==
  data: xyzSensor input double size=[101 2251 3]; groundMask output boolean size=[101 2251]; validMask input boolean size=[101 2251]
function groundMask = Ground_Segmentation(xyzSensor, validMask)
%#codegen
% Ground segmentation on the ORGANIZED, SENSOR-FRAME point cloud.
%
%   xyzSensor  [101 2251 3] double  organized XYZ, sensor frame (NaN = no return)
%   validMask  [101 2251]   boolean finite, non-ego points from LiDAR_Preprocess
%   groundMask [101 2251]   boolean true where the point lies on the ground surface
%
% The range image this algorithm operates on is only defined in the sensor
% frame, so segmentation stays here; the ego-frame cloud is used downstream.

% Algorithm parameters. These are sensor/algorithm properties, NOT scenario
% values, and must stay independent of the loaded scenario.
INITIAL_ELEVATION_ANGLE = 30;   % deg, seed cone for the first ground candidates
ELEVATION_ANGLE_DELTA   = 5;    % deg, tolerance when growing between scan rows

% Exclude invalid and ego-vehicle returns BEFORE building the cloud so they can
% neither seed nor propagate the region growing. NaN is the 'no return'
% encoding that pointCloud and segmentGroundFromLidarData expect.
xyzMasked = xyzSensor;
for k = 1:3
    ch = xyzMasked(:,:,k);
    ch(~validMask) = NaN;
    xyzMasked(:,:,k) = ch;
end

ptCloud = pointCloud(xyzMasked);

groundMask = segmentGroundFromLidarData(ptCloud, ...
    'InitialElevationAngle', INITIAL_ELEVATION_ANGLE, ...
    'ElevationAngleDelta',   ELEVATION_ANGLE_DELTA);

% Guard: never report ground where the preprocess said the point is invalid.
groundMask = groundMask & validMask;

end
